simulink model "ProgettoAO"  (R2021a)
settings: Solver=VariableStepAuto  StartTime=0.0  StopTime=10.0  RelTol=1e-3
values from neighbouring files (symbols this model uses):
  beta = 0.3    [Progetto4c.m]    (also in Progetto_Ada.m)
  den_r = d_r{1}    [Progetto3a.m]    (also in Progetto4c.m; ProgettoGruppoAO.m; Progetto_Ada.m; Prova.m)
  num_r = n_r{1}    [Progetto3a.m]    (also in Progetto4c.m; ProgettoGruppoAO.m; Progetto_Ada.m; Prova.m)
  omega_n = 100    [Progetto3a.m]    (also in Progetto4c.m = 120; ProgettoGruppoAO.m; Progetto_Ada.m = 120; Prova.m)
  W = 5    [Progetto3a.m]    (also in Progetto4c.m = 4; ProgettoGruppoAO.m; Progetto_Ada.m = 4; Prova.m)
settings Model: Creator=Giacomo  LastModifiedBy=Giacomo

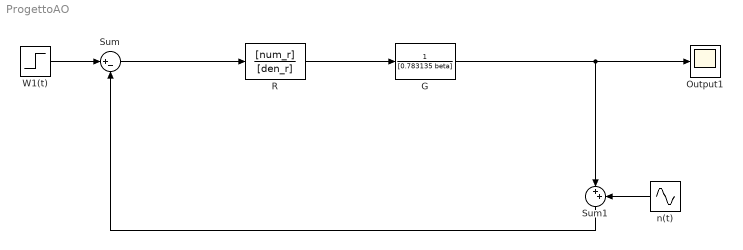
== system ProgettoAO ==
  G : TransferFcn  Denominator=[0.783135 beta]
  Output1 : Scope
  R : TransferFcn  Numerator=[num_r]  Denominator=[den_r]
  Sum : Sum  Inputs=|+-
  Sum1 : Sum  Inputs=|++
  W1(t) : Step  After=W  SampleTime=0
  n(t) : Sin  Amplitude=0.025  Frequency=omega_n  SampleTime=0  VectorParams1D=off
  wires:
  n(t)/1 -> Sum1/2
  R/1 -> G/1
  Sum1/1 -> Sum/2
  Sum/1 -> R/1
  G/1 -> Output1/1, Sum1/1
  W1(t)/1 -> Sum/1
